simulink model "HelicopterLQR"  (R2023a)
settings: Solver=ode4  StartTime=0.0  StopTime=inf  FixedStep=0.1  RelTol=1e-3
values from neighbouring files (symbols this model uses):
  A_c = [0, 0, 1, 0 ... (first row only)    [init_BACKUP.m]
  B_c = [0, 0 ... (first row only)    [init_BACKUP.m]
  C_c = [1,0,0,0 ... (first row only)    [init_BACKUP.m]
  psi_op = pi/2    (= 1.57079632679)    [init_BACKUP.m]
  teta_op = -10*pi/180    (= -0.174532925199)    [init_BACKUP.m]
  V_mp_op = K_yy*m_heli*g*cos(teta_op)*l_cm/(K_yy*K_pp - K_yp*K_py)    [init_BACKUP.m]
  v_my_op = K_yp*V_mp_op/K_yy    [init_BACKUP.m]
  wpsi_op = 0    [init_BACKUP.m]
  wteta_op = 0    [init_BACKUP.m]
undefined symbols (not defined in the file or in its folder): daq, L
libraries: simulink_extras x4, daqlib x2
settings Model: Creator=Jardar Fagerlund  LastModifiedBy=Jardar Fagerlund

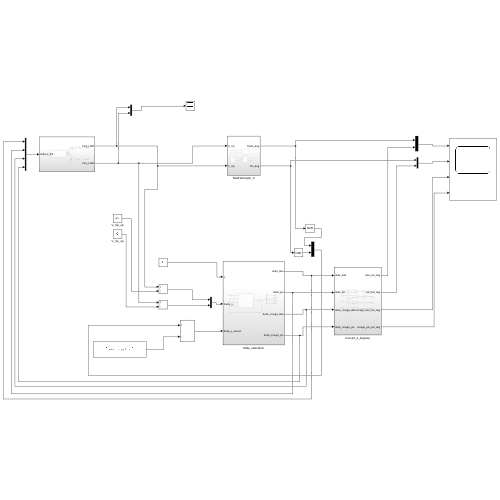
[thumbnail: Simulink's stored preview of the top-level diagram]
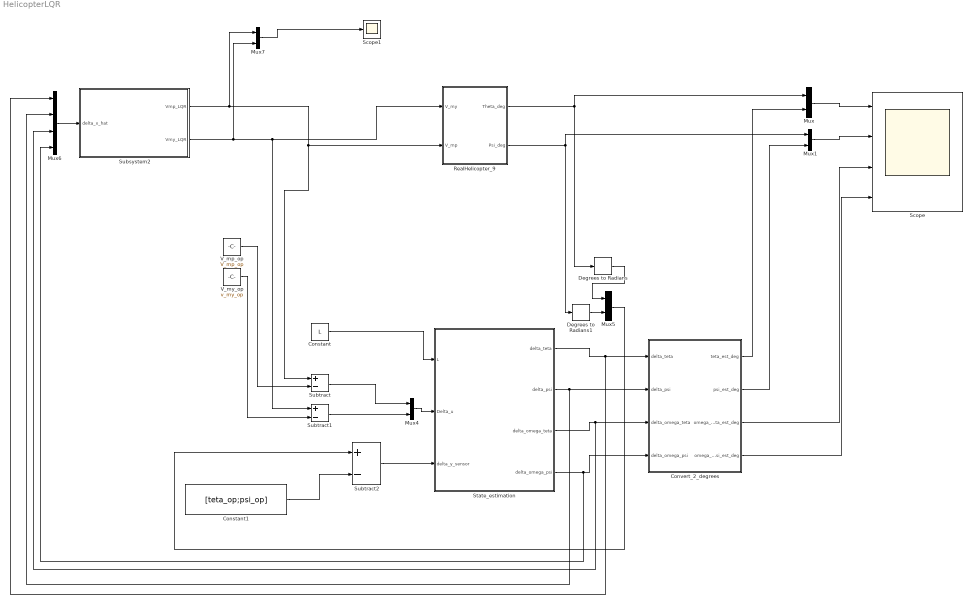
== system HelicopterLQR ==
  Constant : Constant  Value=L
  Constant1 : Constant  Value=[teta_op;psi_op]
  Convert_2_degrees : Subsystem
  Degrees to Radians : simulink_extras/Transformations/Degrees to Radians
  Degrees to Radians1 : simulink_extras/Transformations/Degrees to Radians
  Mux{,1,4..5,7} (5 alike) : Mux  Inputs=2
  Mux6 : Mux
  RealHelicopter_9 : Subsystem
  Scope : Scope  NumInputPorts=4
  Scope1 : Scope
  State_estimation : Subsystem
  Subsystem2 : Subsystem
  Subtract : Sum  Inputs=+-
  Subtract1 : Sum  Inputs=+-
  Subtract2 : Sum  Inputs=+-
  V_mp_op : Constant  Value=V_mp_op
  V_my_op : Constant  Value=v_my_op
  wires:
  Subsystem2/1(Vmp_LQR) -> Mux7/1, Subtract/1, RealHelicopter_9/2(V_mp)
  Subsystem2/2(Vmy_LQR) -> Mux7/2, RealHelicopter_9/1(V_my), Subtract1/1
  RealHelicopter_9/1(Theta_deg) -> Mux/1, Degrees to Radians/1
  RealHelicopter_9/2(Psi_deg) -> Mux1/1, Degrees to Radians1/1
  Mux/1 -> Scope/1
  Mux1/1 -> Scope/2
  Convert_2_degrees/3(omega_teta_est_deg) -> Scope/3
  Convert_2_degrees/4(omega_psi_est_deg) -> Scope/4
  V_my_op/1 -> Subtract1/2
  Constant/1 -> State_estimation/1(L)
  Subtract/1 -> Mux4/1
  Subtract1/1 -> Mux4/2
  Mux4/1 -> State_estimation/2(Delta_u)
  Subtract2/1 -> State_estimation/3(delta_y_sensor)
  Constant1/1 -> Subtract2/2
  Mux5/1 -> Subtract2/1
  V_mp_op/1 -> Subtract/2
  State_estimation/1(delta_teta) -> Mux6/1, Convert_2_degrees/1(delta_teta)
  State_estimation/2(delta_psi) -> Convert_2_degrees/2(delta_psi), Mux6/2
  State_estimation/3(delta_omega_teta) -> Mux6/3, Convert_2_degrees/3(delta_omega_teta)
  State_estimation/4(delta_omega_psi) -> Mux6/4, Convert_2_degrees/4(delta_omega_psi)
  Convert_2_degrees/1(teta_est_deg) -> Mux/2
  Convert_2_degrees/2(psi_est_deg) -> Mux1/2
  Degrees to Radians1/1 -> Mux5/2
  Degrees to Radians/1 -> Mux5/1
  Mux6/1 -> Subsystem2/1(delta_x_hat)
  Mux7/1 -> Scope1/1

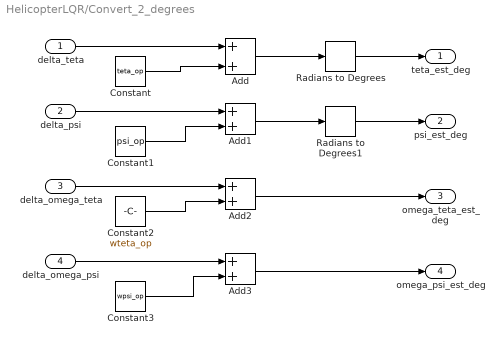
== system HelicopterLQR/Convert_2_degrees ==
  delta_teta : Inport
  delta_psi : Inport  Port=2
  delta_omega_teta : Inport  Port=3
  delta_omega_psi : Inport  Port=4
  Add{,1..3} (4 alike) : Sum
  Constant : Constant  Value=teta_op
  Constant1 : Constant  Value=psi_op
  Constant2 : Constant  Value=wteta_op
  Constant3 : Constant  Value=wpsi_op
  Radians to Degrees : simulink_extras/Transformations/Radians to Degrees
  Radians to Degrees1 : simulink_extras/Transformations/Radians to Degrees
  teta_est_deg : Outport
  psi_est_deg : Outport  Port=2
  omega_teta_est_deg : Outport  Port=3
  omega_psi_est_deg : Outport  Port=4
  wires:
  Add1/1 -> Radians to Degrees1/1
  Add/1 -> Radians to Degrees/1
  delta_teta/1 -> Add/1
  delta_omega_psi/1 -> Add3/1
  delta_omega_teta/1 -> Add2/1
  delta_psi/1 -> Add1/1
  Constant/1 -> Add/2
  Constant1/1 -> Add1/2
  Constant2/1 -> Add2/2
  Constant3/1 -> Add3/2
  Radians to Degrees/1 -> teta_est_deg/1
  Radians to Degrees1/1 -> psi_est_deg/1
  Add3/1 -> omega_psi_est_deg/1
  Add2/1 -> omega_teta_est_deg/1

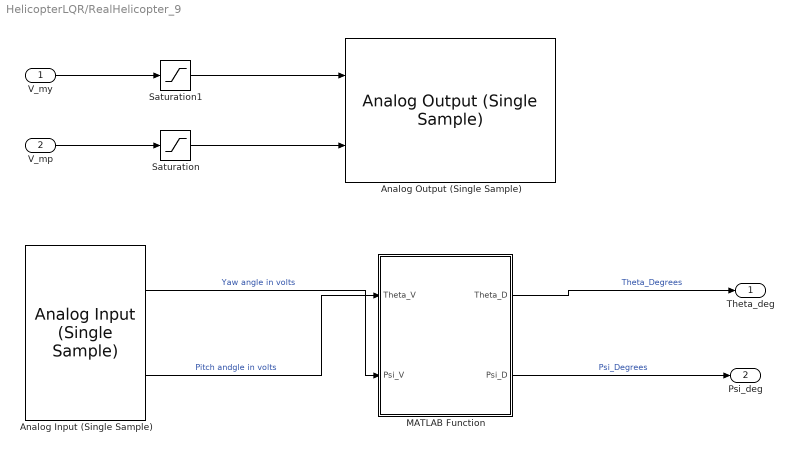
== system HelicopterLQR/RealHelicopter_9 ==
  V_my : Inport
  V_mp : Inport  Port=2
  Analog Input (Single Sample) : daqlib/Analog Input (Single Sample)  DeviceMenu=ni Dev1 (USB-6001)  Device=ni Dev1 (USB-6001)  ObjConstructor=daq.createSession('ni')  BlockSampleTime=0.1  NChannelsSelected=2  Channels=1$ai0$$Dev1$1$1$1$1$#1$ai1$$Dev1$1$1$1$1$#0$ai2$$Dev1$1$1$2$1$#0$ai3$$Dev1$1$1$2$1$#0$ai4$$Dev1$1$1$1$1$#0$ai5$$Dev1$1$1$1$1$#0$ai6$$Dev1$1$1$1$1$#0$ai7$$Dev1$1$1$1$1$#  NPorts=1 per channel  OutputTimestamp=off
  Analog Output (Single Sample) : daqlib/Analog Output (Single Sample)  DeviceMenu=ni Dev1 (USB-6001)  Device=ni Dev1 (USB-6001)  ObjConstructor=daq.createSession('ni')  NChannelsSelected=2  Channels=1$ao0$$Dev1$1$1$N/A$#1$ao1$$Dev1$1$1$N/A$#  NPorts=1 per channel  BlockSampleTime=0.1
  MATLAB Function : MATLAB Function  TreatAsAtomicUnit=on
  Saturation : Saturate  UpperLimit=3  LowerLimit=0
  Saturation1 : Saturate  UpperLimit=3  LowerLimit=0
  Theta_deg : Outport
  Psi_deg : Outport  Port=2
  wires:
  Saturation1/1 -> Analog Output (Single Sample)/1
  Saturation/1 -> Analog Output (Single Sample)/2
  Analog Input (Single Sample)/1 -> MATLAB Function/2(Psi_V)  "Yaw angle in volts"
  Analog Input (Single Sample)/2 -> MATLAB Function/1(Theta_V)  "Pitch andgle in volts"
  MATLAB Function/1(Theta_D) -> Theta_deg/1  "Theta_Degrees"
  MATLAB Function/2(Psi_D) -> Psi_deg/1  "Psi_Degrees"
  V_my/1 -> Saturation1/1
  V_mp/1 -> Saturation/1

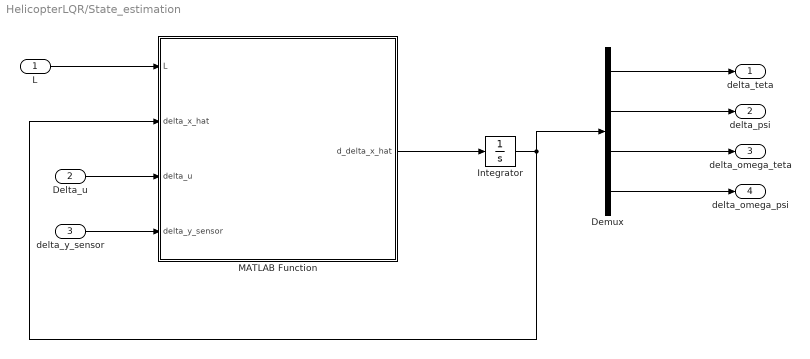
== system HelicopterLQR/State_estimation ==
  L : Inport
  Delta_u : Inport  Port=2
  delta_y_sensor : Inport  Port=3
  Demux : Demux
  Integrator : Integrator  InitialCondition=[-20*pi/180;20*pi/180;0;0];  LimitOutput=on  UpperSaturationLimit=[45*pi/180 - teta_op; pi-psi_op;inf;inf];  LowerSaturationLimit=[-45*pi/180-teta_op; 0-psi_op; -inf;-inf];
  MATLAB Function : MATLAB Function  TreatAsAtomicUnit=on
  delta_teta : Outport
  delta_psi : Outport  Port=2
  delta_omega_teta : Outport  Port=3
  delta_omega_psi : Outport  Port=4
  wires:
  L/1 -> MATLAB Function/1(L)
  MATLAB Function/1(d_delta_x_hat) -> Integrator/1
  Integrator/1 -> MATLAB Function/2(delta_x_hat), Demux/1
  Delta_u/1 -> MATLAB Function/3(delta_u)
  delta_y_sensor/1 -> MATLAB Function/4(delta_y_sensor)
  Demux/4 -> delta_omega_psi/1
  Demux/3 -> delta_omega_teta/1
  Demux/2 -> delta_psi/1
  Demux/1 -> delta_teta/1

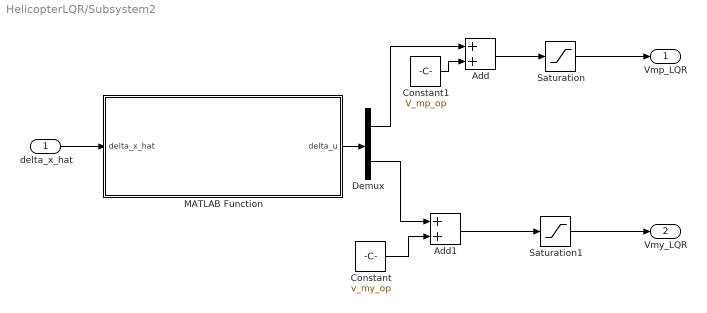
== system HelicopterLQR/Subsystem2 ==
  delta_x_hat : Inport
  Add : Sum
  Add1 : Sum
  Constant : Constant  Value=v_my_op
  Constant1 : Constant  Value=V_mp_op
  Demux : Demux  Outputs=2
  MATLAB Function : MATLAB Function  TreatAsAtomicUnit=on
  Saturation : Saturate  UpperLimit=3  LowerLimit=0
  Saturation1 : Saturate  UpperLimit=3  LowerLimit=0
  Vmp_LQR : Outport
  Vmy_LQR : Outport  Port=2
  wires:
  delta_x_hat/1 -> MATLAB Function/1(delta_x_hat)
  MATLAB Function/1(delta_u) -> Demux/1
  Demux/2 -> Add1/1
  Demux/1 -> Add/1
  Constant/1 -> Add1/2
  Constant1/1 -> Add/2
  Add1/1 -> Saturation1/1
  Add/1 -> Saturation/1
  Saturation/1 -> Vmp_LQR/1
  Saturation1/1 -> Vmy_LQR/1

== matlab function HelicopterLQR/Subsystem2/MATLAB Function ==
  data: delta_x_hat input; delta_u output; K parameter
function delta_u = lqr(delta_x_hat,K)

delta_u = -K*delta_x_hat;

== matlab function HelicopterLQR/State_estimation/MATLAB Function ==
  data: L input; d_delta_x_hat output; delta_x_hat input; delta_u input; delta_y_sensor input; A_c parameter; B_c parameter; C_c parameter
function d_delta_x_hat = StateEstimation(L, delta_x_hat, delta_u, delta_y_sensor, A_c, B_c, C_c)

d_delta_x_hat = A_c*delta_x_hat + B_c*delta_u + L*(delta_y_sensor - C_c*delta_x_hat);

== matlab function HelicopterLQR/RealHelicopter_9/MATLAB Function ==
  data: Theta_V input; Theta_D output; Psi_V input; Psi_D output
function [Theta_D, Psi_D] = VoltageToDegrees(Theta_V, Psi_V)

Theta_D = 90*Theta_V/5 - 45;
Psi_D = 180*Psi_V/5;
